simulink library "rocket_drag_library"  (R2014a)
settings: Solver=ode45  StartTime=0.0  StopTime=10.0  RelTol=1e-3
settings Model: Creator=scorpii  LastModifiedBy=scorpii

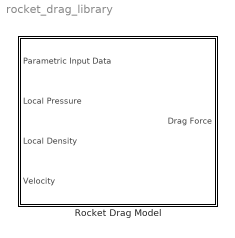
== system rocket_drag_library ==
  Rocket Drag Model : Subsystem

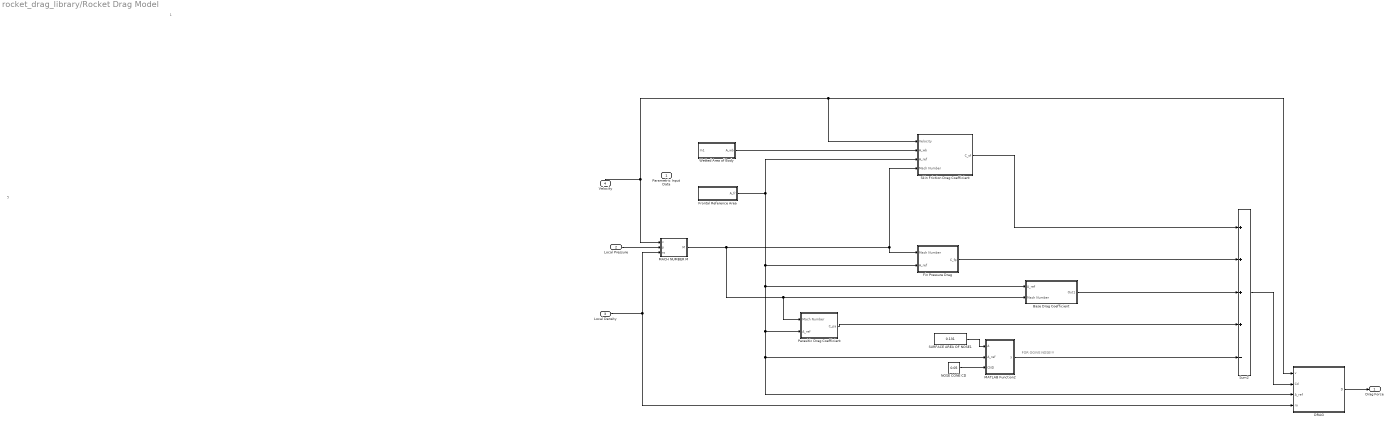
== system rocket_drag_library/Rocket Drag Model ==
  note: 1
  note: 5
  note: FOR OGIVE NOSE!!!
  Parametric Input Data : Inport
  Local Pressure : Inport  Port=2
  Local Density : Inport  Port=3
  Velocity : Inport  Port=4
  Base Drag Coefficient : Subsystem
  DRAG : Subsystem  TreatAsAtomicUnit=on
  Fin Pressure Drag : Subsystem
  Frontal Reference Area : Subsystem
  MACH NUMBER M : Subsystem  TreatAsAtomicUnit=on
  MATLAB Function2 : Subsystem  TreatAsAtomicUnit=on
  NOSE CONE CD : Constant  Value=0.05
  Parasitic Drag Coefficient : Subsystem
  SURFACE AREA OF NOSE1 : Constant  Value=0.131
  Skin Friction Drag Coefficient : Subsystem
  Sum2 : Sum  Inputs=++++-
  Wetted Area of Body : Subsystem
  Drag Force : Outport
  wires:
  Velocity/1 -> MACH NUMBER M/1(v), Skin Friction Drag Coefficient/1(Velocity), DRAG/1(v)
  MACH NUMBER M/1(M) -> Parasitic Drag Coefficient/1(Mach Number), Base Drag Coefficient/2(Mach Number), Skin Friction Drag Coefficient/4(Mach Number), Fin Pressure Drag/1(Mach Number)
  Sum2/1 -> DRAG/2(Cd)
  NOSE CONE CD/1 -> MATLAB Function2/3(CND)
  MATLAB Function2/1(y) -> Sum2/5
  Local Density/1 -> DRAG/4(ro), MACH NUMBER M/3(ro)
  Local Pressure/1 -> MACH NUMBER M/2(p)
  DRAG/1(D) -> Drag Force/1
  SURFACE AREA OF NOSE1/1 -> MATLAB Function2/1(A)
  Frontal Reference Area/1(A_fr) -> Skin Friction Drag Coefficient/3(A_ref), DRAG/3(A_ref), MATLAB Function2/2(A_ref), Parasitic Drag Coefficient/2(A_ref), Base Drag Coefficient/1(A_ref), Fin Pressure Drag/2(A_ref)
  Parasitic Drag Coefficient/1(C_pa) -> Sum2/4
  Base Drag Coefficient/1(Out1) -> Sum2/3
  Fin Pressure Drag/1(C_fp) -> Sum2/2
  Wetted Area of Body/1(A_wb) -> Skin Friction Drag Coefficient/2(A_wb)
  Skin Friction Drag Coefficient/1(C_sf) -> Sum2/1

== system rocket_drag_library/Rocket Drag Model/Base Drag Coefficient ==
  A_ref : Inport
  Mach Number : Inport  Port=2
  BASE DRAG COEF : Subsystem  TreatAsAtomicUnit=on
  Gain1 : Gain
  NORMALIZED BASE DRAG COEF : Subsystem  TreatAsAtomicUnit=on
  OUTER DIAMETER (m)3 : Constant  Value=0.104
  Out1 : Outport
  wires:
  Gain1/1 -> Out1/1
  BASE DRAG COEF/1(C_base) -> NORMALIZED BASE DRAG COEF/1(C_base)
  NORMALIZED BASE DRAG COEF/1(C_base_n) -> Gain1/1
  Mach Number/1 -> BASE DRAG COEF/1(M)
  A_ref/1 -> NORMALIZED BASE DRAG COEF/2(A_ref)
  OUTER DIAMETER (m)3/1 -> NORMALIZED BASE DRAG COEF/3(OD)

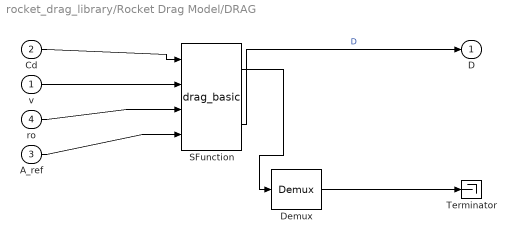
== system rocket_drag_library/Rocket Drag Model/DRAG ==
  v : Inport
  Cd : Inport  Port=2
  A_ref : Inport  Port=3
  ro : Inport  Port=4
  " Demux " : Demux  Outputs=1
  " SFunction " : S-Function  Tag=Stateflow S-Function VELOCITY_MODEL 4  FunctionName=drag_basic  PortCounts=[4 2]  EnableBusSupport=on
  " Terminator " : Terminator
  D : Outport
  wires:
  Cd/1 -> " SFunction "/1
  v/1 -> " SFunction "/2
  ro/1 -> " SFunction "/3
  A_ref/1 -> " SFunction "/4
  " SFunction "/2 -> D/1  "D"
  " Demux "/1 -> " Terminator "/1
  " SFunction "/1 -> " Demux "/1

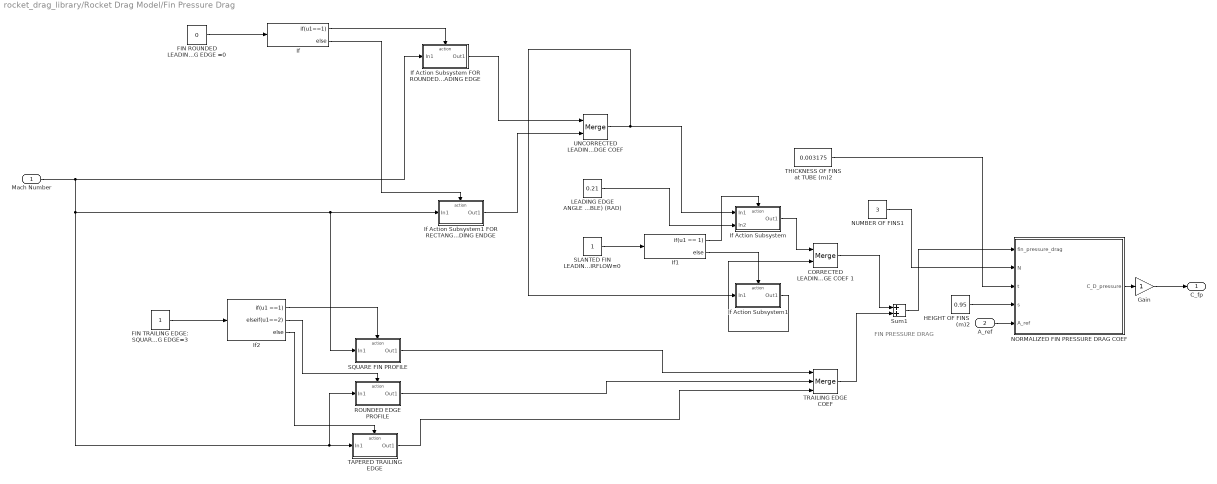
== system rocket_drag_library/Rocket Drag Model/Fin Pressure Drag ==
  note: FIN PRESSURE DRAG
  Mach Number : Inport
  A_ref : Inport  Port=2
  CORRECTED LEADING EDGE COEF 1 : Merge
  FIN ROUNDED LEADING EDGE=1 RECT' LEADING EDGE =0 : Constant  Value=0
  "FIN TRAILING EDGE: SQUARE FIN PROFILE=1 ROUNDED EDGE PROFILE=2 TAPERED TRAILING EDGE=3 " : Constant
  Gain : Gain
  HEIGHT OF FINS (m)2 : Constant  Value=0.95
  If : If  IfExpression=u1==1
  If Action Subsystem : Subsystem  TreatAsAtomicUnit=on
  If Action Subsystem FOR ROUNDED LEADING EDGE : Subsystem  TreatAsAtomicUnit=on
  If Action Subsystem1 : Subsystem  TreatAsAtomicUnit=on
  If Action Subsystem1 FOR RECTANGULAR LEADING ENDGE : Subsystem  TreatAsAtomicUnit=on
  If1 : If  IfExpression=u1 == 1
  If2 : If  IfExpression=u1 ==1  ElseIfExpressions=u1==2
  LEADING EDGE ANGLE (IF APPLICABLE) (RAD) : Constant  Value=0.21
  NORMALIZED FIN PRESSURE DRAG COEF : Subsystem  TreatAsAtomicUnit=on
  NUMBER OF FINS1 : Constant  Value=3
  ROUNDED EDGE PROFILE : Subsystem  TreatAsAtomicUnit=on
  SLANTED FIN LEADING EDGE=1 FIN PERPENDICULAR TO AIRFLOW=0 : Constant
  SQUARE FIN PROFILE : Subsystem  TreatAsAtomicUnit=on
  Sum1 : Sum
  TAPERED TRAILING EDGE : Subsystem  TreatAsAtomicUnit=on
  THICKNESS OF FINS at TUBE (m)2 : Constant  Value=0.003175
  TRAILING EDGE COEF : Merge  Inputs=3
  "UNCORRECTED LEADING EDGE COEF " : Merge
  C_fp : Outport
  wires:
  SLANTED FIN LEADING EDGE=1 FIN PERPENDICULAR TO AIRFLOW=0/1 -> If1/1
  FIN ROUNDED LEADING EDGE=1 RECT' LEADING EDGE =0/1 -> If/1
  LEADING EDGE ANGLE (IF APPLICABLE) (RAD)/1 -> If Action Subsystem/2(In2)
  CORRECTED LEADING EDGE COEF 1/1 -> Sum1/1
  If2/2 -> ROUNDED EDGE PROFILE/Action
  TAPERED TRAILING EDGE/1(Out1) -> TRAILING EDGE COEF/3
  If/1 -> If Action Subsystem FOR ROUNDED LEADING EDGE/Action
  If Action Subsystem FOR ROUNDED LEADING EDGE/1(Out1) -> "UNCORRECTED LEADING EDGE COEF "/1
  Sum1/1 -> NORMALIZED FIN PRESSURE DRAG COEF/1(fin_pressure_drag)
  SQUARE FIN PROFILE/1(Out1) -> TRAILING EDGE COEF/1
  If1/2 -> If Action Subsystem1/Action
  If2/3 -> TAPERED TRAILING EDGE/Action
  Gain/1 -> C_fp/1
  If1/1 -> If Action Subsystem/Action
  If/2 -> If Action Subsystem1 FOR RECTANGULAR LEADING ENDGE/Action
  "UNCORRECTED LEADING EDGE COEF "/1 -> If Action Subsystem1/1(In1), If Action Subsystem/1(In1)
  NORMALIZED FIN PRESSURE DRAG COEF/1(C_D_pressure) -> Gain/1
  If Action Subsystem1 FOR RECTANGULAR LEADING ENDGE/1(Out1) -> "UNCORRECTED LEADING EDGE COEF "/2
  If Action Subsystem/1(Out1) -> CORRECTED LEADING EDGE COEF 1/1
  ROUNDED EDGE PROFILE/1(Out1) -> TRAILING EDGE COEF/2
  TRAILING EDGE COEF/1 -> Sum1/2
  If Action Subsystem1/1(Out1) -> CORRECTED LEADING EDGE COEF 1/2
  "FIN TRAILING EDGE: SQUARE FIN PROFILE=1 ROUNDED EDGE PROFILE=2 TAPERED TRAILING EDGE=3 "/1 -> If2/1
  If2/1 -> SQUARE FIN PROFILE/Action
  HEIGHT OF FINS (m)2/1 -> NORMALIZED FIN PRESSURE DRAG COEF/4(s)
  THICKNESS OF FINS at TUBE (m)2/1 -> NORMALIZED FIN PRESSURE DRAG COEF/3(t)
  Mach Number/1 -> ROUNDED EDGE PROFILE/1(In1), TAPERED TRAILING EDGE/1(In1), SQUARE FIN PROFILE/1(In1), If Action Subsystem1 FOR RECTANGULAR LEADING ENDGE/1(In1), If Action Subsystem FOR ROUNDED LEADING EDGE/1(In1)
  A_ref/1 -> NORMALIZED FIN PRESSURE DRAG COEF/5(A_ref)
  NUMBER OF FINS1/1 -> NORMALIZED FIN PRESSURE DRAG COEF/2(N)

== system rocket_drag_library/Rocket Drag Model/Frontal Reference Area ==
  HEIGHT OF FINS (m) : Constant  Value=0.95
  NUMBER OF FINS : Constant  Value=3
  OUTER DIAMETER (m) : Constant  Value=0.104
  REFERENCE AREA (frontal area) : Subsystem  TreatAsAtomicUnit=on
  THICKNESS OF FINS at TUBE (m) : Constant  Value=0.003175
  A_fr : Outport
  wires:
  REFERENCE AREA (frontal area)/1(A_ref) -> A_fr/1
  NUMBER OF FINS/1 -> REFERENCE AREA (frontal area)/2(N)
  THICKNESS OF FINS at TUBE (m)/1 -> REFERENCE AREA (frontal area)/3(t)
  HEIGHT OF FINS (m)/1 -> REFERENCE AREA (frontal area)/4(s)
  OUTER DIAMETER (m)/1 -> REFERENCE AREA (frontal area)/1(OD)

== system rocket_drag_library/Rocket Drag Model/MACH NUMBER M ==
  v : Inport
  p : Inport  Port=2
  ro : Inport  Port=3
  " Demux " : Demux  Outputs=1
  " SFunction " : S-Function  Tag=Stateflow S-Function VELOCITY_MODEL 15  FunctionName=mach_number  PortCounts=[3 2]  EnableBusSupport=on
  " Terminator " : Terminator
  M : Outport
  wires:
  v/1 -> " SFunction "/1
  p/1 -> " SFunction "/2
  ro/1 -> " SFunction "/3
  " SFunction "/2 -> M/1  "M"
  " Demux "/1 -> " Terminator "/1
  " SFunction "/1 -> " Demux "/1

== system rocket_drag_library/Rocket Drag Model/MATLAB Function2 ==
  A : Inport
  A_ref : Inport  Port=2
  CND : Inport  Port=3
  " Demux " : Demux  Outputs=1
  " SFunction " : S-Function  Tag=Stateflow S-Function VELOCITY_MODEL 32  FunctionName=sf_sfun  PortCounts=[3 2]  EnableBusSupport=on
  " Terminator " : Terminator
  y : Outport
  wires:
  A/1 -> " SFunction "/1
  A_ref/1 -> " SFunction "/2
  CND/1 -> " SFunction "/3
  " SFunction "/2 -> y/1  "y"
  " Demux "/1 -> " Terminator "/1
  " SFunction "/1 -> " Demux "/1

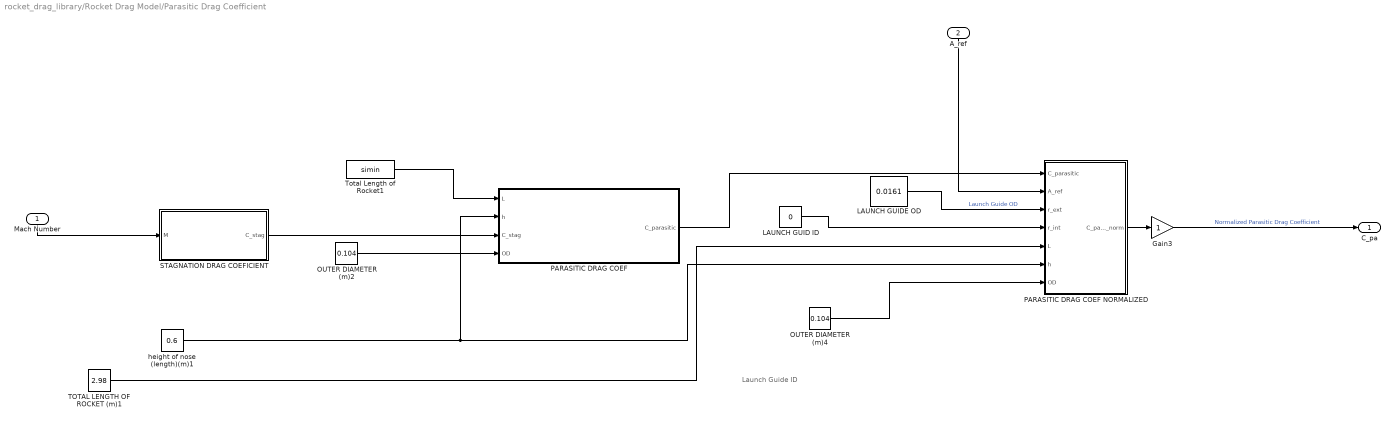
== system rocket_drag_library/Rocket Drag Model/Parasitic Drag Coefficient ==
  note: Launch Guide ID
  Mach Number : Inport
  A_ref : Inport  Port=2
  Gain3 : Gain
  LAUNCH GUID ID : Constant  Value=0
  LAUNCH GUIDE OD : Constant  Value=0.0161
  OUTER DIAMETER (m)2 : Constant  Value=0.104
  OUTER DIAMETER (m)4 : Constant  Value=0.104
  PARASITIC DRAG COEF : Subsystem  TreatAsAtomicUnit=on
  PARASITIC DRAG COEF NORMALIZED : Subsystem  TreatAsAtomicUnit=on
  STAGNATION DRAG COEFICIENT : Subsystem  TreatAsAtomicUnit=on
  TOTAL LENGTH OF ROCKET (m)1 : Constant  Value=2.98
  Total Length of Rocket1 : FromWorkspace  VariableName=simin  SampleTime=0
  height of nose (length)(m)1 : Constant  Value=0.6
  C_pa : Outport
  wires:
  STAGNATION DRAG COEFICIENT/1(C_stag) -> PARASITIC DRAG COEF/3(C_stag)
  Gain3/1 -> C_pa/1  "Normalized Parasitic Drag Coefficient"
  LAUNCH GUIDE OD/1 -> PARASITIC DRAG COEF NORMALIZED/3(r_ext)  "Launch Guide OD"
  Total Length of Rocket1/1 -> PARASITIC DRAG COEF/1(L)
  PARASITIC DRAG COEF/1(C_parasitic) -> PARASITIC DRAG COEF NORMALIZED/1(C_parasitic)
  PARASITIC DRAG COEF NORMALIZED/1(C_parasitic_norm) -> Gain3/1
  LAUNCH GUID ID/1 -> PARASITIC DRAG COEF NORMALIZED/4(r_int)
  A_ref/1 -> PARASITIC DRAG COEF NORMALIZED/2(A_ref)
  Mach Number/1 -> STAGNATION DRAG COEFICIENT/1(M)
  OUTER DIAMETER (m)4/1 -> PARASITIC DRAG COEF NORMALIZED/7(OD)
  TOTAL LENGTH OF ROCKET (m)1/1 -> PARASITIC DRAG COEF NORMALIZED/5(L)
  height of nose (length)(m)1/1 -> PARASITIC DRAG COEF/2(h), PARASITIC DRAG COEF NORMALIZED/6(h)
  OUTER DIAMETER (m)2/1 -> PARASITIC DRAG COEF/4(OD)

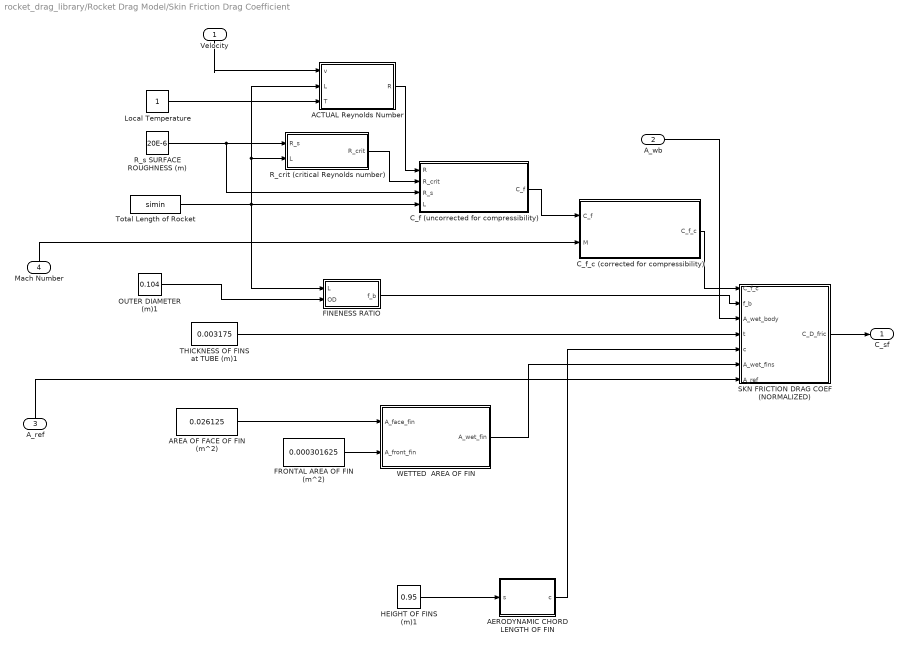
== system rocket_drag_library/Rocket Drag Model/Skin Friction Drag Coefficient ==
  Velocity : Inport
  A_wb : Inport  Port=2
  A_ref : Inport  Port=3
  Mach Number : Inport  Port=4
  ACTUAL Reynolds Number : Subsystem  TreatAsAtomicUnit=on
  AERODYNAMIC CHORD LENGTH OF FIN : Subsystem  TreatAsAtomicUnit=on
  AREA OF FACE OF FIN (m^2) : Constant  Value=0.026125
  C_f (uncorrected for compressibility) : Subsystem  TreatAsAtomicUnit=on
  C_f_c (corrected for compressibility) : Subsystem  TreatAsAtomicUnit=on
  FINENESS RATIO : Subsystem  TreatAsAtomicUnit=on
  FRONTAL AREA OF FIN (m^2) : Constant  Value=0.000301625
  HEIGHT OF FINS (m)1 : Constant  Value=0.95
  "Local Temperature " : Constant
  OUTER DIAMETER (m)1 : Constant  Value=0.104
  R_crit (critical Reynolds number) : Subsystem  TreatAsAtomicUnit=on
  R_s SURFACE ROUGHNESS (m) : Constant  Value=20E-6
  SKN FRICTION DRAG COEF (NORMALIZED) : Subsystem  TreatAsAtomicUnit=on
  THICKNESS OF FINS at TUBE (m)1 : Constant  Value=0.003175
  Total Length of Rocket : FromWorkspace  VariableName=simin  SampleTime=0
  WETTED  AREA OF FIN : Subsystem  TreatAsAtomicUnit=on
  C_sf : Outport
  wires:
  WETTED  AREA OF FIN/1(A_wet_fin) -> SKN FRICTION DRAG COEF (NORMALIZED)/6(A_wet_fins)
  R_s SURFACE ROUGHNESS (m)/1 -> C_f (uncorrected for compressibility)/3(R_s), R_crit (critical Reynolds number)/1(R_s)
  C_f (uncorrected for compressibility)/1(C_f) -> C_f_c (corrected for compressibility)/1(C_f)
  R_crit (critical Reynolds number)/1(R_crit) -> C_f (uncorrected for compressibility)/2(R_crit)
  C_f_c (corrected for compressibility)/1(C_f_c) -> SKN FRICTION DRAG COEF (NORMALIZED)/1(C_f_c)
  ACTUAL Reynolds Number/1(R) -> C_f (uncorrected for compressibility)/1(R)
  FINENESS RATIO/1(f_b) -> SKN FRICTION DRAG COEF (NORMALIZED)/2(f_b)
  AERODYNAMIC CHORD LENGTH OF FIN/1(c) -> SKN FRICTION DRAG COEF (NORMALIZED)/5(c)
  "Local Temperature "/1 -> ACTUAL Reynolds Number/3(T)
  AREA OF FACE OF FIN (m^2)/1 -> WETTED  AREA OF FIN/1(A_face_fin)
  SKN FRICTION DRAG COEF (NORMALIZED)/1(C_D_fric) -> C_sf/1
  FRONTAL AREA OF FIN (m^2)/1 -> WETTED  AREA OF FIN/2(A_front_fin)
  HEIGHT OF FINS (m)1/1 -> AERODYNAMIC CHORD LENGTH OF FIN/1(s)
  Mach Number/1 -> C_f_c (corrected for compressibility)/2(M)
  OUTER DIAMETER (m)1/1 -> FINENESS RATIO/2(OD)
  A_ref/1 -> SKN FRICTION DRAG COEF (NORMALIZED)/7(A_ref)
  Velocity/1 -> ACTUAL Reynolds Number/1(v)
  Total Length of Rocket/1 -> FINENESS RATIO/1(L), ACTUAL Reynolds Number/2(L), R_crit (critical Reynolds number)/2(L), C_f (uncorrected for compressibility)/4(L)
  A_wb/1 -> SKN FRICTION DRAG COEF (NORMALIZED)/3(A_wet_body)
  THICKNESS OF FINS at TUBE (m)1/1 -> SKN FRICTION DRAG COEF (NORMALIZED)/4(t)

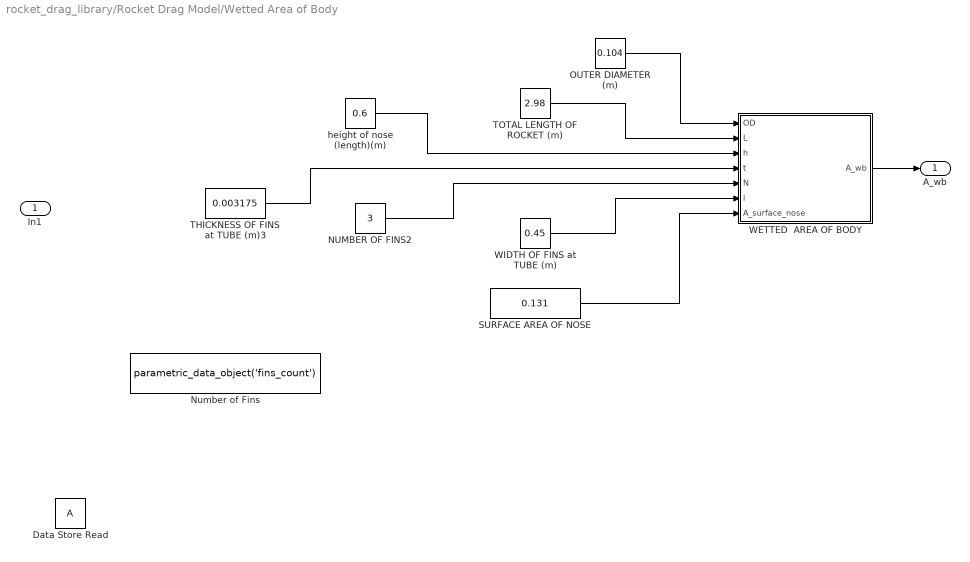
== system rocket_drag_library/Rocket Drag Model/Wetted Area of Body ==
  In1 : Inport
  Data Store Read : DataStoreRead
  NUMBER OF FINS2 : Constant  Value=3
  Number of Fins : FromWorkspace  VariableName=parametric_data_object('fins_count')  SampleTime=0
  OUTER DIAMETER (m) : Constant  Value=0.104
  SURFACE AREA OF NOSE : Constant  Value=0.131
  THICKNESS OF FINS at TUBE (m)3 : Constant  Value=0.003175
  TOTAL LENGTH OF ROCKET (m) : Constant  Value=2.98
  WETTED  AREA OF BODY : Subsystem  TreatAsAtomicUnit=on
  WIDTH OF FINS at TUBE (m) : Constant  Value=0.45
  height of nose (length)(m) : Constant  Value=0.6
  A_wb : Outport
  wires:
  SURFACE AREA OF NOSE/1 -> WETTED  AREA OF BODY/7(A_surface_nose)
  TOTAL LENGTH OF ROCKET (m)/1 -> WETTED  AREA OF BODY/2(L)
  WIDTH OF FINS at TUBE (m)/1 -> WETTED  AREA OF BODY/6(l)
  height of nose (length)(m)/1 -> WETTED  AREA OF BODY/3(h)
  NUMBER OF FINS2/1 -> WETTED  AREA OF BODY/5(N)
  WETTED  AREA OF BODY/1(A_wb) -> A_wb/1
  OUTER DIAMETER (m)/1 -> WETTED  AREA OF BODY/1(OD)
  THICKNESS OF FINS at TUBE (m)3/1 -> WETTED  AREA OF BODY/4(t)

== system rocket_drag_library/Rocket Drag Model/Base Drag Coefficient/BASE DRAG COEF ==
  M : Inport
  " Demux " : Demux  Outputs=1
  " SFunction " : S-Function  Tag=Stateflow S-Function VELOCITY_MODEL 10  FunctionName=sf_sfun  PortCounts=[1 2]  EnableBusSupport=on
  " Terminator " : Terminator
  C_base : Outport
  wires:
  M/1 -> " SFunction "/1
  " SFunction "/2 -> C_base/1  "C_base"
  " Demux "/1 -> " Terminator "/1
  " SFunction "/1 -> " Demux "/1

== system rocket_drag_library/Rocket Drag Model/Base Drag Coefficient/NORMALIZED BASE DRAG COEF ==
  C_base : Inport
  A_ref : Inport  Port=2
  OD : Inport  Port=3
  " Demux " : Demux  Outputs=1
  " SFunction " : S-Function  Tag=Stateflow S-Function VELOCITY_MODEL 23  FunctionName=sf_sfun  PortCounts=[3 2]  EnableBusSupport=on
  " Terminator " : Terminator
  C_base_n : Outport
  wires:
  C_base/1 -> " SFunction "/1
  A_ref/1 -> " SFunction "/2
  OD/1 -> " SFunction "/3
  " SFunction "/2 -> C_base_n/1  "C_base_n"
  " Demux "/1 -> " Terminator "/1
  " SFunction "/1 -> " Demux "/1

== system rocket_drag_library/Rocket Drag Model/Fin Pressure Drag/If Action Subsystem ==
  In1 : Inport
  In2 : Inport  Port=2
  Action Port : ActionPort
  MATLAB Function : Subsystem  TreatAsAtomicUnit=on
  Out1 : Outport
  wires:
  In1/1 -> MATLAB Function/1(in1)
  In2/1 -> MATLAB Function/2(in2)
  MATLAB Function/1(y) -> Out1/1

== system rocket_drag_library/Rocket Drag Model/Fin Pressure Drag/If Action Subsystem FOR ROUNDED LEADING EDGE ==
  In1 : Inport
  Action Port : ActionPort
  MATLAB Function : Subsystem  TreatAsAtomicUnit=on
  Out1 : Outport
  wires:
  In1/1 -> MATLAB Function/1(u)
  MATLAB Function/1(y) -> Out1/1

== system rocket_drag_library/Rocket Drag Model/Fin Pressure Drag/If Action Subsystem1 ==
  In1 : Inport
  Action Port : ActionPort
  Out1 : Outport
  wires:
  In1/1 -> Out1/1

== system rocket_drag_library/Rocket Drag Model/Fin Pressure Drag/If Action Subsystem1 FOR RECTANGULAR LEADING ENDGE ==
  In1 : Inport
  Action Port : ActionPort
  MATLAB Function : Subsystem  TreatAsAtomicUnit=on
  Out1 : Outport
  wires:
  In1/1 -> MATLAB Function/1(M)
  MATLAB Function/1(C_stag) -> Out1/1

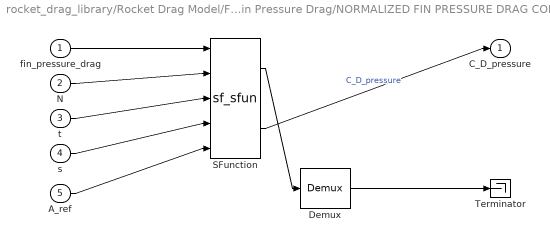
== system rocket_drag_library/Rocket Drag Model/Fin Pressure Drag/NORMALIZED FIN PRESSURE DRAG COEF ==
  fin_pressure_drag : Inport
  N : Inport  Port=2
  t : Inport  Port=3
  s : Inport  Port=4
  A_ref : Inport  Port=5
  " Demux " : Demux  Outputs=1
  " SFunction " : S-Function  Tag=Stateflow S-Function VELOCITY_MODEL 5  FunctionName=sf_sfun  PortCounts=[5 2]  EnableBusSupport=on
  " Terminator " : Terminator
  C_D_pressure : Outport
  wires:
  fin_pressure_drag/1 -> " SFunction "/1
  N/1 -> " SFunction "/2
  t/1 -> " SFunction "/3
  s/1 -> " SFunction "/4
  A_ref/1 -> " SFunction "/5
  " SFunction "/2 -> C_D_pressure/1  "C_D_pressure"
  " Demux "/1 -> " Terminator "/1
  " SFunction "/1 -> " Demux "/1

== system rocket_drag_library/Rocket Drag Model/Fin Pressure Drag/ROUNDED EDGE PROFILE ==
  In1 : Inport
  Action Port : ActionPort
  Gain : Gain  Gain=0.5
  MATLAB Function : Subsystem  TreatAsAtomicUnit=on
  Out1 : Outport
  wires:
  In1/1 -> MATLAB Function/1(M)
  MATLAB Function/1(C_base) -> Gain/1
  Gain/1 -> Out1/1

== system rocket_drag_library/Rocket Drag Model/Fin Pressure Drag/SQUARE FIN PROFILE ==
  In1 : Inport
  Action Port : ActionPort
  MATLAB Function : Subsystem  TreatAsAtomicUnit=on
  Out1 : Outport
  wires:
  In1/1 -> MATLAB Function/1(M)
  MATLAB Function/1(C_base) -> Out1/1

== system rocket_drag_library/Rocket Drag Model/Fin Pressure Drag/TAPERED TRAILING EDGE ==
  In1 : Inport
  Action Port : ActionPort
  Gain : Gain  Gain=0
  Out1 : Outport
  wires:
  In1/1 -> Gain/1
  Gain/1 -> Out1/1

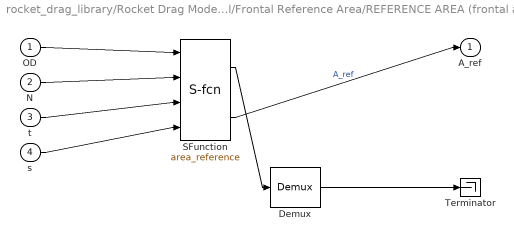
== system rocket_drag_library/Rocket Drag Model/Frontal Reference Area/REFERENCE AREA (frontal area) ==
  OD : Inport
  N : Inport  Port=2
  t : Inport  Port=3
  s : Inport  Port=4
  " Demux " : Demux  Outputs=1
  " SFunction " : S-Function  Tag=Stateflow S-Function VELOCITY_MODEL 9  FunctionName=area_reference  PortCounts=[4 2]  EnableBusSupport=on
  " Terminator " : Terminator
  A_ref : Outport
  wires:
  OD/1 -> " SFunction "/1
  N/1 -> " SFunction "/2
  t/1 -> " SFunction "/3
  s/1 -> " SFunction "/4
  " SFunction "/2 -> A_ref/1  "A_ref"
  " Demux "/1 -> " Terminator "/1
  " SFunction "/1 -> " Demux "/1

== system rocket_drag_library/Rocket Drag Model/Parasitic Drag Coefficient/PARASITIC DRAG COEF ==
  L : Inport
  h : Inport  Port=2
  C_stag : Inport  Port=3
  OD : Inport  Port=4
  " Demux " : Demux  Outputs=1
  " SFunction " : S-Function  Tag=Stateflow S-Function VELOCITY_MODEL 11  FunctionName=coef_drag_parasitic  PortCounts=[4 2]  EnableBusSupport=on
  " Terminator " : Terminator
  C_parasitic : Outport
  wires:
  L/1 -> " SFunction "/1
  h/1 -> " SFunction "/2
  C_stag/1 -> " SFunction "/3
  OD/1 -> " SFunction "/4
  " SFunction "/2 -> C_parasitic/1  "C_parasitic"
  " Demux "/1 -> " Terminator "/1
  " SFunction "/1 -> " Demux "/1

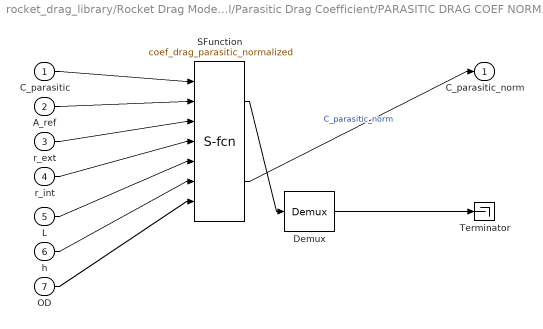
== system rocket_drag_library/Rocket Drag Model/Parasitic Drag Coefficient/PARASITIC DRAG COEF NORMALIZED ==
  C_parasitic : Inport
  A_ref : Inport  Port=2
  r_ext : Inport  Port=3
  r_int : Inport  Port=4
  L : Inport  Port=5
  h : Inport  Port=6
  OD : Inport  Port=7
  " Demux " : Demux  Outputs=1
  " SFunction " : S-Function  Tag=Stateflow S-Function VELOCITY_MODEL 29  FunctionName=coef_drag_parasitic_normalized  PortCounts=[7 2]  EnableBusSupport=on
  " Terminator " : Terminator
  C_parasitic_norm : Outport
  wires:
  C_parasitic/1 -> " SFunction "/1
  A_ref/1 -> " SFunction "/2
  r_ext/1 -> " SFunction "/3
  r_int/1 -> " SFunction "/4
  L/1 -> " SFunction "/5
  h/1 -> " SFunction "/6
  OD/1 -> " SFunction "/7
  " SFunction "/2 -> C_parasitic_norm/1  "C_parasitic_norm"
  " Demux "/1 -> " Terminator "/1
  " SFunction "/1 -> " Demux "/1

== system rocket_drag_library/Rocket Drag Model/Parasitic Drag Coefficient/STAGNATION DRAG COEFICIENT ==
  M : Inport
  " Demux " : Demux  Outputs=1
  " SFunction " : S-Function  Tag=Stateflow S-Function VELOCITY_MODEL 25  FunctionName=coef_drag_stagnation  PortCounts=[1 2]  EnableBusSupport=on
  " Terminator " : Terminator
  C_stag : Outport
  wires:
  M/1 -> " SFunction "/1
  " SFunction "/2 -> C_stag/1  "C_stag"
  " Demux "/1 -> " Terminator "/1
  " SFunction "/1 -> " Demux "/1

== system rocket_drag_library/Rocket Drag Model/Skin Friction Drag Coefficient/ACTUAL Reynolds Number ==
  v : Inport
  L : Inport  Port=2
  T : Inport  Port=3
  " Demux " : Demux  Outputs=1
  " SFunction " : S-Function  Tag=Stateflow S-Function VELOCITY_MODEL 14  FunctionName=sf_sfun  PortCounts=[3 2]  EnableBusSupport=on
  " Terminator " : Terminator
  R : Outport
  wires:
  v/1 -> " SFunction "/1
  L/1 -> " SFunction "/2
  T/1 -> " SFunction "/3
  " SFunction "/2 -> R/1  "R"
  " Demux "/1 -> " Terminator "/1
  " SFunction "/1 -> " Demux "/1

== system rocket_drag_library/Rocket Drag Model/Skin Friction Drag Coefficient/AERODYNAMIC CHORD LENGTH OF FIN ==
  s : Inport
  " Demux " : Demux  Outputs=1
  " SFunction " : S-Function  Tag=Stateflow S-Function VELOCITY_MODEL 19  FunctionName=sf_sfun  PortCounts=[1 2]  EnableBusSupport=on
  " Terminator " : Terminator
  c : Outport
  wires:
  s/1 -> " SFunction "/1
  " SFunction "/2 -> c/1  "c"
  " Demux "/1 -> " Terminator "/1
  " SFunction "/1 -> " Demux "/1

== system rocket_drag_library/Rocket Drag Model/Skin Friction Drag Coefficient/C_f (uncorrected for compressibility) ==
  R : Inport
  R_crit : Inport  Port=2
  R_s : Inport  Port=3
  L : Inport  Port=4
  " Demux " : Demux  Outputs=1
  " SFunction " : S-Function  Tag=Stateflow S-Function VELOCITY_MODEL 13  FunctionName=sf_sfun  PortCounts=[4 2]  EnableBusSupport=on
  " Terminator " : Terminator
  C_f : Outport
  wires:
  R/1 -> " SFunction "/1
  R_crit/1 -> " SFunction "/2
  R_s/1 -> " SFunction "/3
  L/1 -> " SFunction "/4
  " SFunction "/2 -> C_f/1  "C_f"
  " Demux "/1 -> " Terminator "/1
  " SFunction "/1 -> " Demux "/1

== system rocket_drag_library/Rocket Drag Model/Skin Friction Drag Coefficient/C_f_c (corrected for compressibility) ==
  C_f : Inport
  M : Inport  Port=2
  " Demux " : Demux  Outputs=1
  " SFunction " : S-Function  Tag=Stateflow S-Function VELOCITY_MODEL 16  FunctionName=sf_sfun  PortCounts=[2 2]  EnableBusSupport=on
  " Terminator " : Terminator
  C_f_c : Outport
  wires:
  C_f/1 -> " SFunction "/1
  M/1 -> " SFunction "/2
  " SFunction "/2 -> C_f_c/1  "C_f_c"
  " Demux "/1 -> " Terminator "/1
  " SFunction "/1 -> " Demux "/1

== system rocket_drag_library/Rocket Drag Model/Skin Friction Drag Coefficient/FINENESS RATIO ==
  L : Inport
  OD : Inport  Port=2
  " Demux " : Demux  Outputs=1
  " SFunction " : S-Function  Tag=Stateflow S-Function VELOCITY_MODEL 18  FunctionName=sf_sfun  PortCounts=[2 2]  EnableBusSupport=on
  " Terminator " : Terminator
  f_b : Outport
  wires:
  L/1 -> " SFunction "/1
  OD/1 -> " SFunction "/2
  " SFunction "/2 -> f_b/1  "f_b"
  " Demux "/1 -> " Terminator "/1
  " SFunction "/1 -> " Demux "/1

== system rocket_drag_library/Rocket Drag Model/Skin Friction Drag Coefficient/R_crit (critical Reynolds number) ==
  R_s : Inport
  L : Inport  Port=2
  " Demux " : Demux  Outputs=1
  " SFunction " : S-Function  Tag=Stateflow S-Function VELOCITY_MODEL 12  FunctionName=sf_sfun  PortCounts=[2 2]  EnableBusSupport=on
  " Terminator " : Terminator
  R_crit : Outport
  wires:
  R_s/1 -> " SFunction "/1
  L/1 -> " SFunction "/2
  " SFunction "/2 -> R_crit/1  "R_crit"
  " Demux "/1 -> " Terminator "/1
  " SFunction "/1 -> " Demux "/1

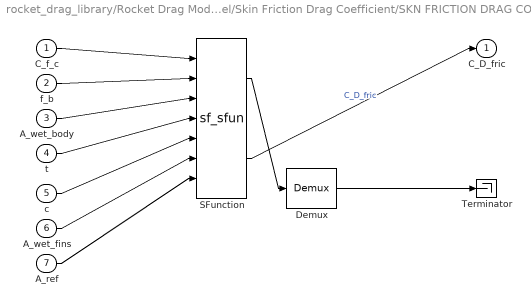
== system rocket_drag_library/Rocket Drag Model/Skin Friction Drag Coefficient/SKN FRICTION DRAG COEF (NORMALIZED) ==
  C_f_c : Inport
  f_b : Inport  Port=2
  A_wet_body : Inport  Port=3
  t : Inport  Port=4
  c : Inport  Port=5
  A_wet_fins : Inport  Port=6
  A_ref : Inport  Port=7
  " Demux " : Demux  Outputs=1
  " SFunction " : S-Function  Tag=Stateflow S-Function VELOCITY_MODEL 20  FunctionName=sf_sfun  PortCounts=[7 2]  EnableBusSupport=on
  " Terminator " : Terminator
  C_D_fric : Outport
  wires:
  C_f_c/1 -> " SFunction "/1
  f_b/1 -> " SFunction "/2
  A_wet_body/1 -> " SFunction "/3
  t/1 -> " SFunction "/4
  c/1 -> " SFunction "/5
  A_wet_fins/1 -> " SFunction "/6
  A_ref/1 -> " SFunction "/7
  " SFunction "/2 -> C_D_fric/1  "C_D_fric"
  " Demux "/1 -> " Terminator "/1
  " SFunction "/1 -> " Demux "/1

== system rocket_drag_library/Rocket Drag Model/Skin Friction Drag Coefficient/WETTED  AREA OF FIN ==
  A_face_fin : Inport
  A_front_fin : Inport  Port=2
  " Demux " : Demux  Outputs=1
  " SFunction " : S-Function  Tag=Stateflow S-Function VELOCITY_MODEL 22  FunctionName=sf_sfun  PortCounts=[2 2]  EnableBusSupport=on
  " Terminator " : Terminator
  A_wet_fin : Outport
  wires:
  A_face_fin/1 -> " SFunction "/1
  A_front_fin/1 -> " SFunction "/2
  " SFunction "/2 -> A_wet_fin/1  "A_wet_fin"
  " Demux "/1 -> " Terminator "/1
  " SFunction "/1 -> " Demux "/1

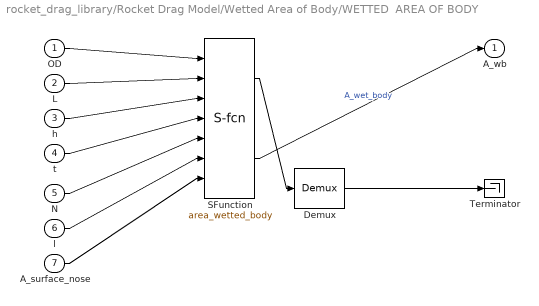
== system rocket_drag_library/Rocket Drag Model/Wetted Area of Body/WETTED  AREA OF BODY ==
  OD : Inport
  L : Inport  Port=2
  h : Inport  Port=3
  t : Inport  Port=4
  N : Inport  Port=5
  l : Inport  Port=6
  A_surface_nose : Inport  Port=7
  " Demux " : Demux  Outputs=1
  " SFunction " : S-Function  Tag=Stateflow S-Function VELOCITY_MODEL 21  FunctionName=area_wetted_body  PortCounts=[7 2]  EnableBusSupport=on
  " Terminator " : Terminator
  A_wb : Outport
  wires:
  OD/1 -> " SFunction "/1
  L/1 -> " SFunction "/2
  h/1 -> " SFunction "/3
  t/1 -> " SFunction "/4
  N/1 -> " SFunction "/5
  l/1 -> " SFunction "/6
  A_surface_nose/1 -> " SFunction "/7
  " SFunction "/2 -> A_wb/1  "A_wet_body"
  " Demux "/1 -> " Terminator "/1
  " SFunction "/1 -> " Demux "/1

== system rocket_drag_library/Rocket Drag Model/Fin Pressure Drag/If Action Subsystem/MATLAB Function ==
  in1 : Inport
  in2 : Inport  Port=2
  " Demux " : Demux  Outputs=1
  " SFunction " : S-Function  Tag=Stateflow S-Function VELOCITY_MODEL 8  FunctionName=sf_sfun  PortCounts=[2 2]  EnableBusSupport=on
  " Terminator " : Terminator
  y : Outport
  wires:
  in1/1 -> " SFunction "/1
  in2/1 -> " SFunction "/2
  " SFunction "/2 -> y/1  "y"
  " Demux "/1 -> " Terminator "/1
  " SFunction "/1 -> " Demux "/1

== system rocket_drag_library/Rocket Drag Model/Fin Pressure Drag/If Action Subsystem FOR ROUNDED LEADING EDGE/MATLAB Function ==
  u : Inport
  " Demux " : Demux  Outputs=1
  " SFunction " : S-Function  Tag=Stateflow S-Function VELOCITY_MODEL 26  FunctionName=sf_sfun  PortCounts=[1 2]  EnableBusSupport=on
  " Terminator " : Terminator
  y : Outport
  wires:
  u/1 -> " SFunction "/1
  " SFunction "/2 -> y/1  "y"
  " Demux "/1 -> " Terminator "/1
  " SFunction "/1 -> " Demux "/1

== system rocket_drag_library/Rocket Drag Model/Fin Pressure Drag/If Action Subsystem1 FOR RECTANGULAR LEADING ENDGE/MATLAB Function ==
  M : Inport
  " Demux " : Demux  Outputs=1
  " SFunction " : S-Function  Tag=Stateflow S-Function VELOCITY_MODEL 27  FunctionName=sf_sfun  PortCounts=[1 2]  EnableBusSupport=on
  " Terminator " : Terminator
  C_stag : Outport
  wires:
  M/1 -> " SFunction "/1
  " SFunction "/2 -> C_stag/1  "C_stag"
  " Demux "/1 -> " Terminator "/1
  " SFunction "/1 -> " Demux "/1

== system rocket_drag_library/Rocket Drag Model/Fin Pressure Drag/ROUNDED EDGE PROFILE/MATLAB Function ==
  M : Inport
  " Demux " : Demux  Outputs=1
  " SFunction " : S-Function  Tag=Stateflow S-Function VELOCITY_MODEL 28  FunctionName=sf_sfun  PortCounts=[1 2]  EnableBusSupport=on
  " Terminator " : Terminator
  C_base : Outport
  wires:
  M/1 -> " SFunction "/1
  " SFunction "/2 -> C_base/1  "C_base"
  " Demux "/1 -> " Terminator "/1
  " SFunction "/1 -> " Demux "/1

== system rocket_drag_library/Rocket Drag Model/Fin Pressure Drag/SQUARE FIN PROFILE/MATLAB Function ==
  M : Inport
  " Demux " : Demux  Outputs=1
  " SFunction " : S-Function  Tag=Stateflow S-Function VELOCITY_MODEL 24  FunctionName=sf_sfun  PortCounts=[1 2]  EnableBusSupport=on
  " Terminator " : Terminator
  C_base : Outport
  wires:
  M/1 -> " SFunction "/1
  " SFunction "/2 -> C_base/1  "C_base"
  " Demux "/1 -> " Terminator "/1
  " SFunction "/1 -> " Demux "/1
